simulink model "SLWOUP"  (R2022b)
settings: configuration reference "SharedConfig" (kept outside this file)
values from neighbouring files (symbols this model uses):
  CanPwrPwmEna_C = 0.0    [SLWOUP.sldd]
  DT_SLWOUP_C = 0.1    [SLWOUP.sldd]
  GreenLedDialEna_C = 0.0    [SLWOUP.sldd]
  GreenLedDialVal_C = 0.0    [SLWOUP.sldd]
  GreenLedIvt_C = 1.0    [SLWOUP.sldd]
  InPwrPwmEna_C = 0.0    [SLWOUP.sldd]
  LedOffTi_C = 0.5    [SLWOUP.sldd]
  LedPlsCtDft_C = 1.0    [SLWOUP.sldd]
  LedPlsCtOpenLoop_C = 2.0    [SLWOUP.sldd]
  LedPlsCtSpdCtl_C = 4.0    [SLWOUP.sldd]
  LedPlsCtTqCtl_C = 3.0    [SLWOUP.sldd]
  McuData2DaDialEna_C = 0.0    [SLWOUP.sldd]
  McuData2DaDialVal_CA : value not decoded    [SLWOUP.sldd]
  MtrPwrPwmEna_C = 0.0    [SLWOUP.sldd]
  PhaPwmEnaDialEna_C = 1.0    [SLWOUP.sldd]
  PhaPwmEnaDialVal_C = 0.0    [SLWOUP.sldd]
  PlsOffTi_C = 0.2    [SLWOUP.sldd]
  PlsOnTi_C = 0.2    [SLWOUP.sldd]
  RedLedDialEna_C = 0.0    [SLWOUP.sldd]
  RedLedDialVal_C = 0.0    [SLWOUP.sldd]
  RedLedIvt_C = 1.0    [SLWOUP.sldd]
  ResolverExctEna_C = 0.0    [SLWOUP.sldd]
  SwPwrPwmEna_C = 0.0    [SLWOUP.sldd]
  YellowLedCmd_C = 1.0    [SLWOUP.sldd]
undefined symbols (not defined in the file or in its folder): DRIVEMODE, slcm
libraries: canmsglib x1, simulink x1
Description:
  | Converts engineering unit signals into raw outputs for the slow task rate.
settings Model: DataDictionary=SLWOUP.sldd  Creator=Kevin  LastModifiedBy=Max Kolesnikov
settings ConfigSetRef: SourceName=SharedConfig

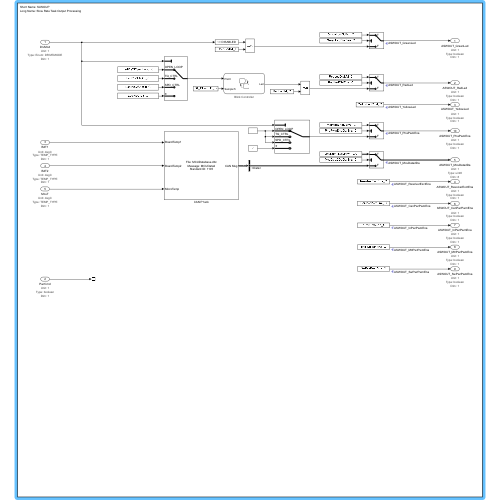
[thumbnail: Simulink's stored preview of the top-level diagram]
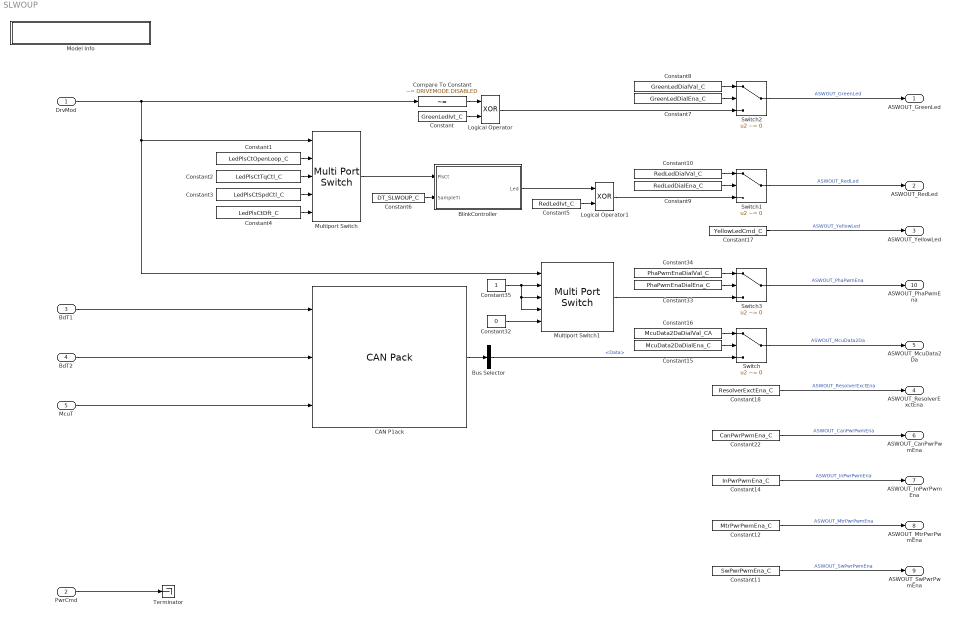
== system SLWOUP ==
  DrvMod : Inport  OutDataTypeStr=Enum: DRIVEMODE  Unit=1  PortDimensions=1
      settings: AttributesFormatString=|
      | Unit: %<Unit>
      | Type: %<OutDataTypeStr>
      | Dim: %<PortDimensions>
  PwrCmd : Inport  Port=2  OutDataTypeStr=boolean  Unit=1  PortDimensions=1
      settings: AttributesFormatString=|
      | Unit: %<Unit>
      | Type: %<OutDataTypeStr>
      | Dim: %<PortDimensions>
  BdT1 : Inport  Port=3  OutDataTypeStr=TEMP_TYPE  Unit=degC  PortDimensions=1
      settings: AttributesFormatString=|
      | Unit: %<Unit>
      | Type: %<OutDataTypeStr>
      | Dim: %<PortDimensions>
  BdT2 : Inport  Port=4  OutDataTypeStr=TEMP_TYPE  Unit=degC  PortDimensions=1
      settings: AttributesFormatString=|
      | Unit: %<Unit>
      | Type: %<OutDataTypeStr>
      | Dim: %<PortDimensions>
  McuT : Inport  Port=5  OutDataTypeStr=TEMP_TYPE  Unit=degC  PortDimensions=1
      settings: AttributesFormatString=|
      | Unit: %<Unit>
      | Type: %<OutDataTypeStr>
      | Dim: %<PortDimensions>
  BlinkController : Stateflow chart  Description=Blink Controller  TreatAsAtomicUnit=on
      settings: AttributesFormatString=%<Description>
  Bus Selector : BusSelector  OutputSignals=Data
  CAN P1ack : canmsglib/CAN Pack  CANdbFile=C:\MKSTechRepos\P2319\p2319asw01\asw\lib\MCUDatabase.dbc  MsgList=MCUData2  MsgName=MCUData2  MsgIDType=Standard (11-bit identifier)  MsgIdentifier=1105  MsgLength=8  Remote=off  ApplyMinMax=off  BusOutput=on  SignalInfo={'BoardTemp1','0','8','LE','unsigned','Standard','0','1','-40','-40','215';'BoardTemp2','8','8','LE','unsigned','Standard','0','1','-40','-40','215';'MicroTemp','16','8','LE','unsigned','Standard','0','1','-40','-40','215'}
      settings: LibrarySourceBlock=embeddedtargetslib/Host Communication/CAN Pack  DataFormat=CANdb specified signals
  Compare To Constant : simulink/Logic and Bit Operations/Compare To Constant  relop=~=  const=DRIVEMODE.DISABLED  OutDataTypeStr=boolean
  Constant : Constant  Value=GreenLedIvt_C
  Constant1 : Constant  Value=LedPlsCtOpenLoop_C
  Constant10 : Constant  Value=RedLedDialVal_C
  Constant11 : Constant  Value=SwPwrPwmEna_C
  Constant12 : Constant  Value=MtrPwrPwmEna_C
  Constant14 : Constant  Value=InPwrPwmEna_C
  Constant15 : Constant  Value=McuData2DaDialEna_C
  Constant16 : Constant  Value=McuData2DaDialVal_CA
  Constant17 : Constant  Value=YellowLedCmd_C
  Constant18 : Constant  Value=ResolverExctEna_C
  Constant2 : Constant  Value=LedPlsCtTqCtl_C
  Constant22 : Constant  Value=CanPwrPwmEna_C
  Constant3 : Constant  Value=LedPlsCtSpdCtl_C
  Constant32 : Constant  Value=0  OutDataTypeStr=boolean
  Constant33 : Constant  Value=PhaPwmEnaDialEna_C
  Constant34 : Constant  Value=PhaPwmEnaDialVal_C
  Constant35 : Constant  OutDataTypeStr=boolean
  Constant4 : Constant  Value=LedPlsCtDft_C
  Constant5 : Constant  Value=RedLedIvt_C
  Constant6 : Constant  Value=DT_SLWOUP_C
  Constant7 : Constant  Value=GreenLedDialEna_C
  Constant8 : Constant  Value=GreenLedDialVal_C
  Constant9 : Constant  Value=RedLedDialEna_C
  Logical Operator : Logic  Operator=XOR  AllPortsSameDT=off  OutDataTypeStr=boolean
  Logical Operator1 : Logic  Operator=XOR  AllPortsSameDT=off  OutDataTypeStr=boolean
  Model Info : Subsystem  LoadFcn=slcm LoadBlock;  InitFcn=slcm('UpdateAllCMBlocksInThisModelInit')  mask(CMBlock){Frame=off, DisplayStringWithTags=|, MaskDisplayString=Short Name: SLWOUP\nLong Name: Slow Rate Task Output Processing, HorizontalTextAlignment=Left, LeftAlignmentValue=0.02}
      mask DisplayStringWithTags=|
      | Short Name: %<ModelName>
      | Long Name: Slow Rate Task Output Processing
      mask prompts: Frame "Simulink:masks:Frame_MP"; DisplayStringWithTags "Simulink:masks:DisplayStringWithTags_MP"; MaskDisplayString "Simulink:masks:MaskDisplayString_MP"; HorizontalTextAlignment "Simulink:masks:HorizontalTextAlignment_MP"; LeftAlignmentValue "Simulink:masks:LeftAlignmentValue_MP"
      mask help: Simulink:masks:CMBlock_MD
      settings: CopyFcn=slcm CopyBlock;  DeleteFcn=slcm Cancel;  PostSaveFcn=slcm('UpdateAllCMBlocksInThisModel')  NameChangeFcn=slcm Rename;  OpenFcn=slcm
      mask Display: text(slResolve(LeftAlignmentValue, gcbh), 0.5, MaskDisplayString, 'HorizontalAlignment', HorizontalTextAlignment)
  Multiport Switch : MultiPortSwitch  DataPortOrder=Specify indices  DataPortIndices={DRIVEMODE.OPEN_LOOP,DRIVEMODE.TQ_CTRL,DRIVEMODE.SPD_CTRL}  DataPortForDefault=Additional data port  DiagnosticForDefault=None  SaturateOnIntegerOverflow=off  InputSameDT=off
  Multiport Switch1 : MultiPortSwitch  DataPortOrder=Specify indices  DataPortIndices={DRIVEMODE.OPEN_LOOP,DRIVEMODE.TQ_CTRL,DRIVEMODE.SPD_CTRL}  DataPortForDefault=Additional data port  DiagnosticForDefault=None  SaturateOnIntegerOverflow=off  InputSameDT=off
  Switch{,1..3} (4 alike) : Switch  Criteria=u2 ~= 0  SaturateOnIntegerOverflow=off  InputSameDT=off
  Terminator : Terminator
  ASWOUT_GreenLed : Outport  OutDataTypeStr=boolean  Unit=1  PortDimensions=1
      settings: AttributesFormatString=|
      | Unit: %<Unit>
      | Type: %<OutDataTypeStr>
      | Dim: %<PortDimensions>
  ASWOUT_RedLed : Outport  Port=2  OutDataTypeStr=boolean  Unit=1  PortDimensions=1
      settings: AttributesFormatString=|
      | Unit: %<Unit>
      | Type: %<OutDataTypeStr>
      | Dim: %<PortDimensions>
  ASWOUT_YellowLed : Outport  Port=3  OutDataTypeStr=boolean  Unit=1  PortDimensions=1
      settings: AttributesFormatString=|
      | Unit: %<Unit>
      | Type: %<OutDataTypeStr>
      | Dim: %<PortDimensions>
  ASWOUT_ResolverExctEna : Outport  Port=4  OutDataTypeStr=boolean  Unit=1  PortDimensions=1
      settings: AttributesFormatString=|
      | Unit: %<Unit>
      | Type: %<OutDataTypeStr>
      | Dim: %<PortDimensions>
  ASWOUT_McuData2Da : Outport  Port=5  OutDataTypeStr=uint8  Unit=1  PortDimensions=8
      settings: AttributesFormatString=|
      | Unit: %<Unit>
      | Type: %<OutDataTypeStr>
      | Dim: %<PortDimensions>
  ASWOUT_CanPwrPwmEna : Outport  Port=6  OutDataTypeStr=boolean  Unit=1  PortDimensions=1
      settings: AttributesFormatString=|
      | Unit: %<Unit>
      | Type: %<OutDataTypeStr>
      | Dim: %<PortDimensions>
  ASWOUT_InPwrPwmEna : Outport  Port=7  OutDataTypeStr=boolean  Unit=1  PortDimensions=1
      settings: AttributesFormatString=|
      | Unit: %<Unit>
      | Type: %<OutDataTypeStr>
      | Dim: %<PortDimensions>
  ASWOUT_MtrPwrPwmEna : Outport  Port=8  OutDataTypeStr=boolean  Unit=1  PortDimensions=1
      settings: AttributesFormatString=|
      | Unit: %<Unit>
      | Type: %<OutDataTypeStr>
      | Dim: %<PortDimensions>
  ASWOUT_SwPwrPwmEna : Outport  Port=9  OutDataTypeStr=boolean  Unit=1  PortDimensions=1
      settings: AttributesFormatString=|
      | Unit: %<Unit>
      | Type: %<OutDataTypeStr>
      | Dim: %<PortDimensions>
  ASWOUT_PhaPwmEna : Outport  Port=10  OutDataTypeStr=boolean  Unit=1  PortDimensions=1
      settings: AttributesFormatString=|
      | Unit: %<Unit>
      | Type: %<OutDataTypeStr>
      | Dim: %<PortDimensions>
  wires:
  Switch1/1 -> ASWOUT_RedLed/1  "ASWOUT_RedLed"
  DrvMod/1 -> Multiport Switch1/1, Multiport Switch/1, Compare To Constant/1
  Multiport Switch/1 -> BlinkController/1(PlsCt)
  Compare To Constant/1 -> Logical Operator/1
  Constant/1 -> Logical Operator/2
  Switch2/1 -> ASWOUT_GreenLed/1  "ASWOUT_GreenLed"
  Constant1/1 -> Multiport Switch/2
  Constant2/1 -> Multiport Switch/3
  Constant3/1 -> Multiport Switch/4
  Constant4/1 -> Multiport Switch/5
  Constant5/1 -> Logical Operator1/2
  BlinkController/1(Led) -> Logical Operator1/1
  Constant6/1 -> BlinkController/2(SampleTi)
  Constant8/1 -> Switch2/1
  Constant7/1 -> Switch2/2
  Constant9/1 -> Switch1/2
  Constant10/1 -> Switch1/1
  Logical Operator1/1 -> Switch1/3
  Logical Operator/1 -> Switch2/3
  Bus Selector/1 -> Switch/3  "<Data>"
  Constant15/1 -> Switch/2
  Constant16/1 -> Switch/1
  CAN P1ack/1 -> Bus Selector/1
  Switch/1 -> ASWOUT_McuData2Da/1  "ASWOUT_McuData2Da"
  BdT1/1 -> CAN P1ack/1
  BdT2/1 -> CAN P1ack/2
  McuT/1 -> CAN P1ack/3
  Constant17/1 -> ASWOUT_YellowLed/1  "ASWOUT_YellowLed"
  Constant18/1 -> ASWOUT_ResolverExctEna/1  "ASWOUT_ResolverExctEna"
  Constant22/1 -> ASWOUT_CanPwrPwmEna/1  "ASWOUT_CanPwrPwmEna"
  PwrCmd/1 -> Terminator/1
  Constant14/1 -> ASWOUT_InPwrPwmEna/1  "ASWOUT_InPwrPwmEna"
  Constant12/1 -> ASWOUT_MtrPwrPwmEna/1  "ASWOUT_MtrPwrPwmEna"
  Constant11/1 -> ASWOUT_SwPwrPwmEna/1  "ASWOUT_SwPwrPwmEna"
  Constant32/1 -> Multiport Switch1/5
  Multiport Switch1/1 -> Switch3/3
  Constant34/1 -> Switch3/1
  Constant33/1 -> Switch3/2
  Switch3/1 -> ASWOUT_PhaPwmEna/1  "ASWOUT_PhaPwmEna"
  Constant35/1 -> Multiport Switch1/4, Multiport Switch1/3, Multiport Switch1/2

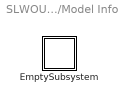
== system SLWOUP/Model Info ==
  EmptySubsystem : Subsystem

== system SLWOUP/Model Info/EmptySubsystem ==

== stateflow chart SLWOUP/BlinkController ==
  state PULSE
    state PULSE_ON
      en:
      PlsOnTmr = 0;
      du:
      PlsOnTmr = PlsOnTmr + SampleTi;
      Led = true;
    state PULSE_OFF
      en:
      PlsOffTmr = 0;
      PlsCtr = PlsCtr + 1;
      du:
      PlsOffTmr = PlsOffTmr + SampleTi;
      Led = false;
    (default) -> PULSE_ON
    PULSE_ON -> PULSE_OFF : [PlsOnTmr >= PlsOnTi_C]
    PULSE_OFF -> PULSE_ON : [PlsOffTmr >= PlsOffTi_C]
  state OFF
    en:
    OffTmr = 0;
    PlsCtr = 0;
    du:
    OffTmr = OffTmr + SampleTi;
    Led = false;
  (default) -> OFF
  OFF -> PULSE : [OffTmr >= LedOffTi_C && ...
      | PlsCtr < PlsCt]
  PULSE -> OFF : [PlsCtr >= PlsCt]
  data: PlsCt input; OffTmr local single; PlsOnTmr local single; PlsOffTmr local single; Led output boolean; PlsCtr local uint8; PlsOnTi_C parameter; PlsOffTi_C parameter; LedOffTi_C parameter; SampleTi input
